simulink model "suspensionsimulink"  (R2018b)
settings: Solver=VariableStepAuto  StartTime=0.0  StopTime=20  RelTol=1e-3
undefined symbols (not defined in the file): A, B, C, k
libraries: simulink x1
settings Model: Creator=ASUS  LastModifiedBy=ASUS

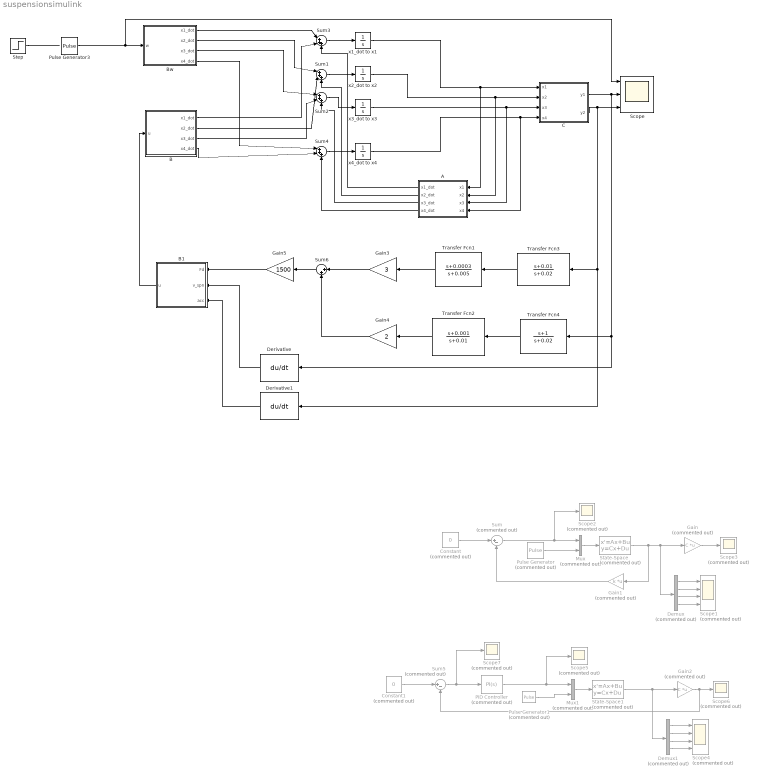
== system suspensionsimulink ==
  A : MATLAB Function  TreatAsAtomicUnit=on
  B : MATLAB Function  TreatAsAtomicUnit=on
  B1 : MATLAB Function  TreatAsAtomicUnit=on
  Bw : MATLAB Function  TreatAsAtomicUnit=on
  C : MATLAB Function  TreatAsAtomicUnit=on
  Constant : Constant  Commented=on  Value=0
  Constant1 : Constant  Commented=on  Value=0
  Demux : Demux  Commented=on
  Demux1 : Demux  Commented=on
  Derivative : Derivative
  Derivative1 : Derivative
  Gain : Gain  Commented=on  Gain=C  Multiplication=Matrix(K*u)
  Gain1 : Gain  Commented=on  Gain=k  Multiplication=Matrix(K*u)
  Gain2 : Gain  Commented=on  Gain=C  Multiplication=Matrix(K*u)
  Gain3 : Gain  Gain=3
  Gain4 : Gain  Gain=2
  Gain5 : Gain  Gain=1500
  Mux : Mux  Commented=on  Inputs=2
  Mux1 : Mux  Commented=on  Inputs=2
  PID Controller : simulink/Continuous/PID Controller  Commented=on  Controller=PI  Form=Parallel  TimeDomain=Continuous-time  SampleTime=-1  IntegratorMethod=Forward Euler  FilterMethod=Forward Euler  ControllerParametersSource=internal  P=1  I=100  D=0  UseFilter=on  N=100  TunerSelectOption=Transfer Function Based (PID Tuner App)  InitialConditionSource=internal  InitialConditionForIntegrator=0  InitialConditionForFilter=0  DifferentiatorICPrevScaledInput=0  ExternalReset=none  TrackingMode=off  Kt=1  LimitOutput=off  UpperSaturationLimit=inf  LowerSaturationLimit=-inf  LinearizeAsGain=on  AntiWindupMode=none  Kb=1  POutMin=[]  POutMax=[]  IOutMin=[]  IOutMax=[]  DOutMin=[]  DOutMax=[]  NOutMin=[]  NOutMax=[]  SumOutMin=[]  SumOutMax=[]  SaturationOutMin=[]  SaturationOutMax=[]  PParamMin=[]  PParamMax=[]  IParamMin=[]  IParamMax=[]  DParamMin=[]  DParamMax=[]  NParamMin=[]  NParamMax=[]  KbParamMin=[]  KbParamMax=[]  KtParamMin=[]  KtParamMax=[]  KbOutMin=[]  KbOutMax=[]  KtOutMin=[]  KtOutMax=[]  IntegratorOutMin=[]  IntegratorOutMax=[]  FilterOutMin=[]  FilterOutMax=[]  SumI1OutMin=[]  SumI1OutMax=[]  SumI2OutMin=[]  SumI2OutMax=[]  SumI3OutMin=[]  SumI3OutMax=[]  SumI4OutMin=[]  SumI4OutMax=[]  SumDOutMin=[]  SumDOutMax=[]  DifferentiatorOutMin=[]  DifferentiatorOutMax=[]  FilterDiffOutCoefMin=[]  FilterDiffOutCoefMax=[]  ReciprocalOutMin=[]  ReciprocalOutMax=[]  SumDenOutMin=[]  SumDenOutMax=[]  SumNumOutMin=[]  SumNumOutMax=[]  DivideOutMin=[]  DivideOutMax=[]  IntegratorContinuousStateAttributes=''  IntegratorStateMustResolveToSignalObject=off  IntegratorRTWStateStorageClass=Auto  FilterContinuousStateAttributes=''  FilterStateMustResolveToSignalObject=off  FilterRTWStateStorageClass=Auto  ParallelPVariant=InternalParameters  IdealPVariant=Disabled  IVariant=InternalParameters  DVariant=Disabled  IntegratorVariant=Continuous  SatVariant=Disabled  AWVariant=Passthrough  PCopyVariant=Disabled  TRVariant=Disabled  FdbkBlocksVariant=Forward  IdealPFdbkVariant=Disabled  SatFdbkVariant=Disabled  DerivativeFilterVariant=Disabled  NVariant=Disabled  NCopyVariant=Disabled_SignalSpec  FilterICVariant=Disabled  IntegratorICVariant=InternalICs  ExternalResetVariant=Disabled  TRSumVariant=Passthrough  SumFdbkVariant=Disabled  SumVariant=Sum_PI
  Pulse Generator : DiscretePulseGenerator  Commented=on  PulseType=Time based  Period=15  PulseWidth=50
  Pulse Generator1 : DiscretePulseGenerator  Commented=on  PulseType=Time based  Period=15  PulseWidth=50
  Pulse Generator3 : DiscretePulseGenerator  PulseType=Time based  Amplitude=2  Period=15  PulseWidth=15
  Scope : Scope  NumInputPorts=3
  Scope1 : Scope  Commented=on  NumInputPorts=4
  Scope{2..3,5..7} (5 alike) : Scope  Commented=on
  Scope4 : Scope  Commented=on  NumInputPorts=4
  State-Space : StateSpace  Commented=on  A=A  B=B  C=eye(4)  D=zeros(4,2)  InitialCondition=0
  State-Space1 : StateSpace  Commented=on  A=A  B=B  C=eye(4)  D=zeros(4,2)  InitialCondition=0
  Step : Step  SampleTime=0
  Sum : Sum  Commented=on  Inputs=|+-
  Sum{1..4} (4 alike) : Sum  Inputs=|+++
  Sum5 : Sum  Commented=on  Inputs=|+-
  Sum6 : Sum  Inputs=|++
  Transfer Fcn1 : TransferFcn  Numerator=[1 0.0003]  Denominator=[1 0.005]
  Transfer Fcn2 : TransferFcn  Numerator=[1 0.001]  Denominator=[1 0.01]
  Transfer Fcn3 : TransferFcn  Numerator=[1 0.01]  Denominator=[1 0.02]
  Transfer Fcn4 : TransferFcn  Numerator=[1 1]  Denominator=[1 0.02]
  x1_dot to x1 : Integrator  InitialCondition=0.001
  x2_dot to x2 : Integrator  InitialCondition=0.001
  x3_dot to x3 : Integrator  InitialCondition=0.001
  x4_dot to x4 : Integrator  InitialCondition=0.001
  wires:
  B/1(x1_dot) -> Sum3/2
  Bw/1(x1_dot) -> Sum3/1
  A/1(x1_dot) -> Sum3/3
  Sum3/1 -> x1_dot to x1/1
  Bw/2(x2_dot) -> Sum1/1
  B/2(x2_dot) -> Sum1/2
  A/2(x2_dot) -> Sum1/3
  Sum1/1 -> x2_dot to x2/1
  Bw/3(x3_dot) -> Sum2/1
  B/3(x3_dot) -> Sum2/2
  A/3(x3_dot) -> Sum2/3
  Sum2/1 -> x3_dot to x3/1
  Bw/4(x4_dot) -> Sum4/1
  B/4(x4_dot) -> Sum4/2
  A/4(x4_dot) -> Sum4/3
  Sum4/1 -> x4_dot to x4/1
  x1_dot to x1/1 -> C/1(x1), A/1(x1)
  x2_dot to x2/1 -> A/2(x2), C/2(x2)
  x3_dot to x3/1 -> A/3(x3), C/3(x3)
  x4_dot to x4/1 -> C/4(x4), A/4(x4)
  C/2(y2) -> Derivative1/1, Transfer Fcn3/1, Scope/3
  C/1(y1) -> Transfer Fcn4/1, Derivative/1, Scope/2
  Step/1 -> ?
  Mux/1 -> State-Space/1
  Pulse Generator/1 -> Mux/2
  State-Space/1 -> Gain1/1, Demux/1, Gain/1
  Demux/1 -> Scope1/1
  Demux/2 -> Scope1/2
  Demux/3 -> Scope1/3
  Demux/4 -> Scope1/4
  Sum/1 -> Scope2/1, Mux/1
  Constant/1 -> Sum/1
  Gain1/1 -> Sum/2
  Gain/1 -> Scope3/1
  Gain2/1 -> Scope6/1, Sum5/2
  Constant1/1 -> Sum5/1
  Sum5/1 -> Scope7/1, PID Controller/1
  Demux1/4 -> Scope4/4
  Demux1/3 -> Scope4/3
  Demux1/2 -> Scope4/2
  Demux1/1 -> Scope4/1
  State-Space1/1 -> Gain2/1, Demux1/1
  Pulse Generator1/1 -> Mux1/2
  Mux1/1 -> State-Space1/1
  PID Controller/1 -> Scope5/1, Mux1/1
  Transfer Fcn3/1 -> Transfer Fcn1/1
  Transfer Fcn4/1 -> Transfer Fcn2/1
  Transfer Fcn1/1 -> Gain3/1
  Transfer Fcn2/1 -> Gain4/1
  Gain3/1 -> Sum6/1
  Gain4/1 -> Sum6/2
  Sum6/1 -> Gain5/1
  Gain5/1 -> B1/1(Fd)
  Derivative/1 -> B1/2(v_spn)
  Derivative1/1 -> B1/3(acc)
  B1/1(u) -> B/1(u)
  Pulse Generator3/1 -> Scope/1, Bw/1(w)

== matlab function suspensionsimulink/B ==
  data: x1_dot output; x2_dot output; x3_dot output; u input; x4_dot output
function [x1_dot, x2_dot, x3_dot, x4_dot]= fcn(u)


Ms=504.5;
Mu=62;

x1_dot=0;
x2_dot=0;
x3_dot=-1/Ms;
x4_dot=-1/Mu;

== matlab function suspensionsimulink/Bw ==
  data: x1_dot output; x2_dot output; x3_dot output; w input; x4_dot output
function [x1_dot, x2_dot, x3_dot, x4_dot]= fcn(w)

x1_dot=0;
x2_dot=-w;
x3_dot=0;
x4_dot=0;

== matlab function suspensionsimulink/A ==
  data: x1_dot output; x2_dot output; x3_dot output; x1 input; x4_dot output; x2 input; x3 input; x4 input
function [x1_dot, x2_dot, x3_dot, x4_dot]= fcn(x1,x2,x3,x4)


Ms=504.5;
Mu=62;
Ks=13100;
Kt=252000;
Cs=400;

x1_dot=x3-x4;
x2_dot=x4;
x3_dot=(-Ks/Ms).*x1 + (-Cs/Ms).*x3 + (Cs/Ms).*x4;
x4_dot=+ (-Ks/Mu).*x1 + (-Kt/Mu).*x2 + (Cs/Mu).*x3 + (-Cs/Mu).*x4;

== matlab function suspensionsimulink/C ==
  data: y1 output; y2 output; x1 input; x2 input; x3 input; x4 input
function [y1,y2]= fcn(x1, x2, x3, x4)


y1=x1;
y2=x3;

== matlab function suspensionsimulink/B1 ==
  data: u output; Fd input; v_spn input; acc input
function u = fcn(Fd,v_spn,acc)

if acc>0
    b=[-165.66 114.63 0.85 -7.39 -0.02 0.29 -8.16e-6 -5.9e-3 5.15e-6 5.65e-5 -3.37e-8 -2.05e-7];
    c=[-535.57 530.84 86.52 -21.73 -4.69 0.64 0.11 -0.01 -1.2e-3 8.34e-5 4.63e-6 -2.69e-7];
    temp1=0;
    temp2=0;
    for i=1:12
        temp1=temp1+b(i).*(v_spn).^(i-1);
        temp2=temp2+c(i).*(v_spn).^(i-1);
    end
    u=(Fd - temp1)/(temp2);
elseif acc<0
    b=[-91.80 121.49 -6.95 -7.06 0.45 0.26 -0.01 -5.1e-3 1.34e-4 4.71e-5 -5.51e-7 -1.68e-7];
    c=[473.89 560.46 -76.17 -26.41 4.01 0.89 -0.09 -0.02 9.98e-4 1.49e-4 -3.96e-6 -5.32e-7];
    temp1=0;
    temp2=0;
    for i=1:12
        temp1=temp1+b(i).*(v_spn).^(i-1);
        temp2=temp2+c(i).*(v_spn).^(i-1);
    end
    u=(Fd - temp1)/(temp2);
else
    u=0;

end
